simulink model "DC_MOTOR_Speed_PID"  (R2018a)
settings: Solver=VariableStepAuto  StartTime=0.0  StopTime=80  RelTol=1e-3
model workspace (MAT data in the model file):
  B = 3.84248890607e-23
  J = 0.000220045119023
  K = 0.0137288693481
  L = 0.11377733063
  R = 0.6
libraries: simulink_extras x2, simulink x1
settings Model: Creator=Hazem Elwakeel  LastModifiedBy=Hazem Elwakeel

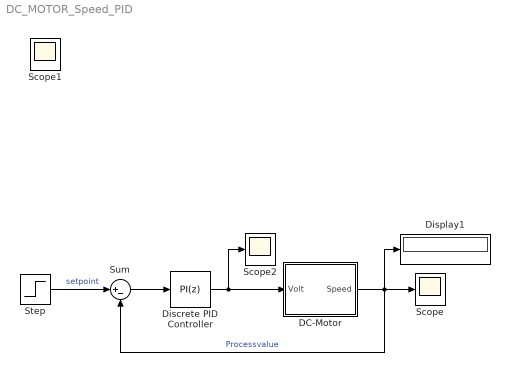
== system DC_MOTOR_Speed_PID ==
  "DC-Motor " : Subsystem
  Discrete PID Controller : simulink/Continuous/PID Controller  Controller=PI  TimeDomain=Discrete-time  SampleTime=0.1  IntegratorMethod=Forward Euler  FilterMethod=Forward Euler  Form=Parallel  UseFilter=off  ControllerParametersSource=internal  P=0.0153213698814719  I=0.0270991729044818  D=0.0122705485184341  N=100  InitialConditionSource=internal  InitialConditionForIntegrator=0  InitialConditionForFilter=0  ExternalReset=none  LimitOutput=on  UpperSaturationLimit=12  LowerSaturationLimit=0  LinearizeAsGain=off  AntiWindupMode=none  Kb=1  TrackingMode=off  Kt=1  PParamMin=[]  PParamMax=[]  IParamMin=[]  IParamMax=[]  DParamMin=[]  DParamMax=[]  NParamMin=[]  NParamMax=[]  KbParamMin=[]  KbParamMax=[]  KtParamMin=[]  KtParamMax=[]  POutMin=[]  POutMax=[]  IOutMin=[]  IOutMax=[]  DOutMin=[]  DOutMax=[]  NOutMin=[]  NOutMax=[]  KbOutMin=[]  KbOutMax=[]  KtOutMin=[]  KtOutMax=[]  IntegratorOutMin=[]  IntegratorOutMax=[]  FilterOutMin=[]  FilterOutMax=[]  SumOutMin=[]  SumOutMax=[]  SumI1OutMin=[]  SumI1OutMax=[]  SumI2OutMin=[]  SumI2OutMax=[]  SumI3OutMin=[]  SumI3OutMax=[]  SumDOutMin=[]  SumDOutMax=[]  SaturationOutMin=[]  SaturationOutMax=[]  IntegratorContinuousStateAttributes=''  IntegratorStateMustResolveToSignalObject=off  IntegratorRTWStateStorageClass=Auto  FilterContinuousStateAttributes=''  FilterStateMustResolveToSignalObject=off  FilterRTWStateStorageClass=Auto  DifferentiatorICPrevScaledInput=0  DifferentiatorOutMin=[]  DifferentiatorOutMax=[]  FilterDiffOutCoefMin=[]  FilterDiffOutCoefMax=[]  SumDenOutMin=[]  SumDenOutMax=[]  SumNumOutMin=[]  SumNumOutMax=[]  ReciprocalOutMin=[]  ReciprocalOutMax=[]  DivideOutMin=[]  DivideOutMax=[]  TunerSelectOption=Transfer Function Based (PID Tuner App)
  Display1 : Display
  Scope : Scope
  Scope2 : Scope
  Step : Step  After=800  SampleTime=0.5
  Sum : Sum  Inputs=|+-
  Scope1 : Scope
  wires:
  Sum/1 -> Discrete PID Controller/1
  "DC-Motor "/1("Speed ") -> Scope/1, Display1/1, Sum/2  "Processvalue"
  Step/1 -> Sum/1  "setpoint"
  Discrete PID Controller/1 -> Scope2/1, "DC-Motor "/1(Volt)

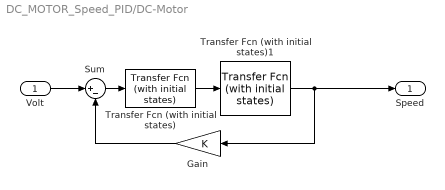
== system DC_MOTOR_Speed_PID/DC-Motor  ==
  Volt : Inport
  Gain : Gain  Gain=K
  Sum : Sum  Inputs=|+-
  Transfer Fcn (with initial states) : simulink_extras/Additional Linear/Transfer Fcn (with initial states)  N=[K]  D="[J  B]"  X0=.5
  Transfer Fcn (with initial states)1 : simulink_extras/Additional Linear/Transfer Fcn (with initial states)  N=[1]  D="[L  R]"  X0=.5
  "Speed " : Outport
  wires:
  Transfer Fcn (with initial states)/1 -> Transfer Fcn (with initial states)1/1
  Gain/1 -> Sum/2
  Transfer Fcn (with initial states)1/1 -> "Speed "/1, Gain/1
  Sum/1 -> Transfer Fcn (with initial states)/1
  Volt/1 -> Sum/1
